simulink model "lib_external"  (Simulink 8.7)
settings: Solver=VariableStepAuto  StartTime=0.0  StopTime=10.0  RelTol=1e-3
settings Model: Creator=pfj01  LastModifiedBy=pfj01
settings DataIOCC: LimitDataPoints=off  SaveFormat=Dataset  SaveOutput=off  SaveTime=off
settings DebuggingCC: UnderspecifiedInitializationDetection=Simplified  MergeDetectMultiDrivingBlocksExec=error
settings HardwareCC: ProdBitPerPointer=64  ProdLargestAtomicFloat=Float  ProdIntDivRoundTo=Zero  ProdEndianess=LittleEndian  ProdWordSize=64  ProdHWDeviceType=Intel->x86-64 (Windows64)
settings ModelReferenceCC: PropagateSignalLabelsOutOfModel=on
settings ConfigComp: CovModelRefEnable=off

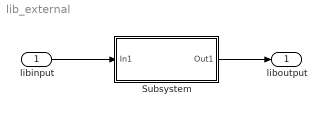
== system lib_external ==
  libinput : Inport  OutDataTypeStr=double  PortDimensions=1  SampleTime=0
  Subsystem : Subsystem
  liboutput : Outport  OutDataTypeStr=double  PortDimensions=1  SampleTime=0
  wires:
  libinput/1 -> Subsystem/1(In1)
  Subsystem/1(Out1) -> liboutput/1

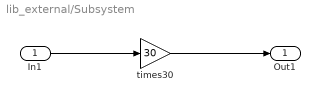
== system lib_external/Subsystem ==
  In1 : Inport
  times30 : Gain  Gain=30
  Out1 : Outport
  wires:
  times30/1 -> Out1/1
  In1/1 -> times30/1
